simulink model "Vehicle"  (R2020a)
settings: Solver=VariableStepAuto  StartTime=0.0  StopTime=10.0  RelTol=1e-3
model workspace (MAT data in the model file):
  VEH.Mass = 330
  VEH.StaticNormalFrontLoad.FR = 74.25
  VEH.StaticNormalFrontLoad.FL = 74.25
  VEH.StaticNormalRearLoad.RR = 90.75
  VEH.StaticNormalRearLoad.RL = 90.75
  VEH.WheelBase = 1.575
  VEH.FrontAxlePositionfromCG = 0.847
  VEH.RearAxlePositionfromCG = 0.693
  VEH.HeightCG = 0.277
  VEH.FrontalArea = 1.435
  VEH.DragCoefficient = 0.33
  VEH.NumberOfWheelsPerAxle = 2
  VEH.Thread.FR = 1.705
  VEH.Thread.RR = 1.705
  VEH.PitchMomentInertia = 206
  VEH.RollMomentInertia = 206.613792
  VEH.YawMomentInertia = 206.613792
  VEH.SteeringRatio = 5.2
  VEH.TrackWidth = 1.2
  VEH.SprungMass = 290
  VEH.InitialLongPosition = 0
  VEH.InitialLatPosition = 0
  VEH.InitialVertPosition = 0
  VEH.InitialRollAngle = 0
  VEH.InitialPitchAngle = 0
  VEH.InitialYawAngle = 0
  VEH.InitialLongVel = 0
  VEH.InitialLatVel = 0
  VEH.InitialVertVel = 0
  VEH.InitialRollRate = 0
  VEH.InitialPitchRate = 0
  VEH.InitialYawRate = 0
  VEH.LongitudinalDragCoefficient = 1.06
  VEH.LongitudinalLCoefficient = -2.05
settings Model: Creator=Administrator  LastModifiedBy=Administrator

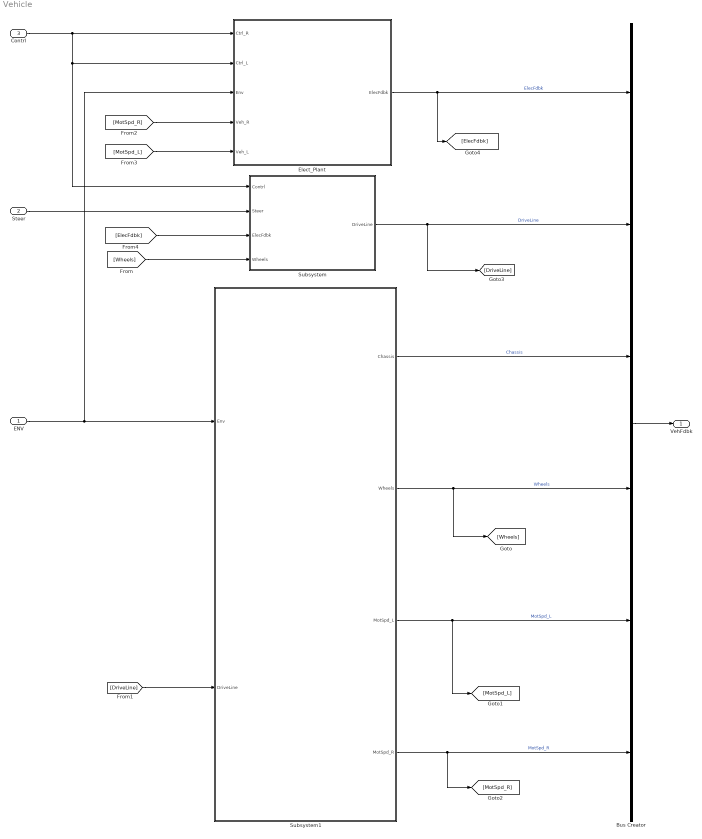
== system Vehicle ==
  ENV : Inport
  Steer : Inport  Port=2
  Contrl : Inport  Port=3
  Bus Creator : BusCreator  Inputs=6
  Elect_Plant : Subsystem
  Subsystem : Subsystem
  Subsystem1 : Subsystem
  VehFdbk : Outport  SignalName=VehFdbk
  wires:
  Elect_Plant/1(ElecFdbk) -> [ElecFdbk], Bus Creator/1  "ElecFdbk"
  Contrl/1 -> Elect_Plant/2(Ctrl_L), Subsystem/1(Contrl), Elect_Plant/1(Ctrl_R)
  Subsystem/1(DriveLine) -> [DriveLine], Bus Creator/2  "DriveLine"
  Subsystem1/1(Chassis) -> Bus Creator/3  "Chassis"
  Subsystem1/2(Wheels) -> [Wheels], Bus Creator/4  "Wheels"
  Subsystem1/3(MotSpd_L) -> [MotSpd_L], Bus Creator/5  "MotSpd_L"
  Subsystem1/4(MotSpd_R) -> [MotSpd_R], Bus Creator/6  "MotSpd_R"
  Bus Creator/1 -> VehFdbk/1
  [MotSpd_R] -> Elect_Plant/4(Veh_R)
  [MotSpd_L] -> Elect_Plant/5(Veh_L)
  Steer/1 -> Subsystem/2(Steer)
  [ElecFdbk] -> Subsystem/3(ElecFdbk)
  [Wheels] -> Subsystem/4(Wheels)
  ENV/1 -> Elect_Plant/3(Env), Subsystem1/1(Env)
  [DriveLine] -> Subsystem1/2(DriveLine)

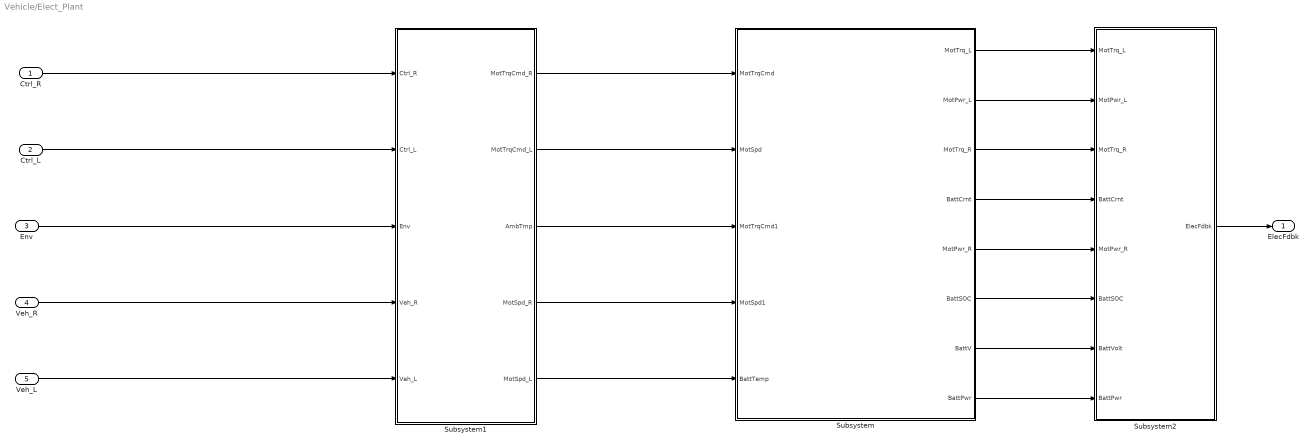
== system Vehicle/Elect_Plant ==
  Ctrl_R : Inport
  Ctrl_L : Inport  Port=2
  Env : Inport  Port=3
  Veh_R : Inport  Port=4
  Veh_L : Inport  Port=5
  Subsystem : Subsystem
  Subsystem1 : Subsystem
  Subsystem2 : Subsystem
  ElecFdbk : Outport
  wires:
  Subsystem1/4(MotSpd_R) -> Subsystem/4(MotSpd1)
  Subsystem1/1(MotTrqCmd_R) -> Subsystem/1(MotTrqCmd)
  Subsystem1/2(MotTrqCmd_L) -> Subsystem/2(MotSpd)
  Subsystem1/3(AmbTmp) -> Subsystem/3(MotTrqCmd1)
  Subsystem1/5(MotSpd_L) -> Subsystem/5(BattTemp)
  Veh_L/1 -> Subsystem1/5(Veh_L)
  Ctrl_R/1 -> Subsystem1/1(Ctrl_R)
  Ctrl_L/1 -> Subsystem1/2(Ctrl_L)
  Env/1 -> Subsystem1/3(Env)
  Veh_R/1 -> Subsystem1/4(Veh_R)
  Subsystem/1(MotTrq_L) -> Subsystem2/1(MotTrq_L)
  Subsystem/2(MotPwr_L) -> Subsystem2/2(MotPwr_L)
  Subsystem/3(MotTrq_R) -> Subsystem2/3(MotTrq_R)
  Subsystem/4(BattCrnt) -> Subsystem2/4(BattCrnt)
  Subsystem/5(MotPwr_R) -> Subsystem2/5(MotPwr_R)
  Subsystem/6(BattSOC) -> Subsystem2/6(BattSOC)
  Subsystem/7(BattV) -> Subsystem2/7(BattVolt)
  Subsystem/8(BattPwr) -> Subsystem2/8(BattPwr)
  Subsystem2/1(ElecFdbk) -> ElecFdbk/1

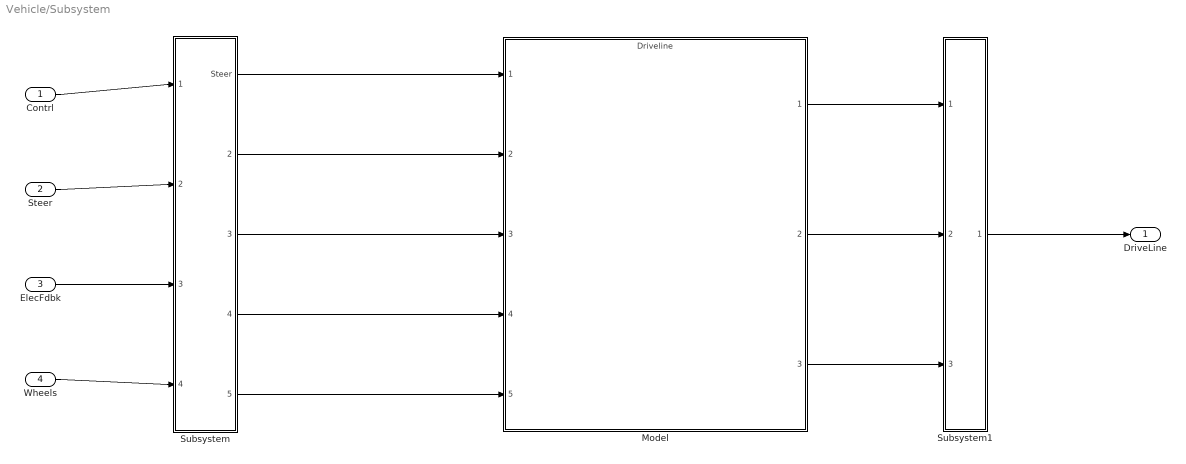
== system Vehicle/Subsystem ==
  Contrl : Inport
  Steer : Inport  Port=2
  ElecFdbk : Inport  Port=3
  Wheels : Inport  Port=4
  Model : ModelReference  ModelNameDialog=Driveline.slx  SimulationMode=Normal  ModelReferenceVersion=1.211
  Subsystem : Subsystem
  Subsystem1 : Subsystem
  DriveLine : Outport
  wires:
  Contrl/1 -> Subsystem/1(Contrl)
  Subsystem/1(Steer) -> Model/1
  Subsystem/2(MotTrq_L) -> Model/2
  Subsystem/3(MotTrq_R) -> Model/3
  Subsystem/4(PrsCmd) -> Model/4
  Subsystem/5(Omega) -> Model/5
  Steer/1 -> Subsystem/2(SteerCmd)
  Wheels/1 -> Subsystem/4(Wheels)
  ElecFdbk/1 -> Subsystem/3(ElecFdbk)
  Model/1 -> Subsystem1/1(WhlAng)
  Model/2 -> Subsystem1/2(AxlTrq)
  Model/3 -> Subsystem1/3(BrkPrs)
  Subsystem1/1(DriverLine) -> DriveLine/1

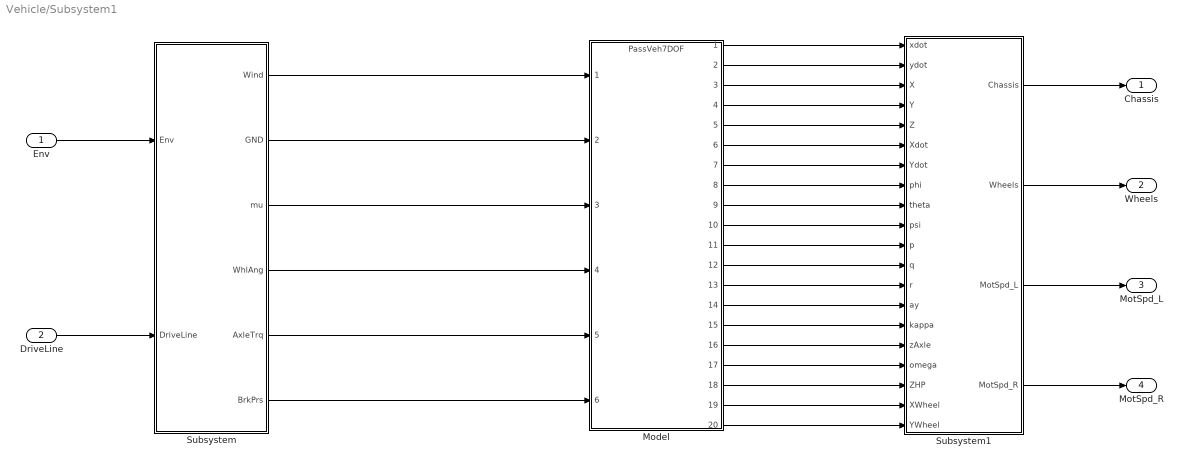
== system Vehicle/Subsystem1 ==
  Env : Inport
  DriveLine : Inport  Port=2
  Model : ModelReference  ModelNameDialog=PassVeh7DOF.slx  SimulationMode=Normal  ModelReferenceVersion=1.128
  Subsystem : Subsystem
  Subsystem1 : Subsystem
  Chassis : Outport
  Wheels : Outport  Port=2
  MotSpd_L : Outport  Port=3
  MotSpd_R : Outport  Port=4
  wires:
  Env/1 -> Subsystem/1(Env)
  Subsystem/1(Wind) -> Model/1
  Subsystem/2(GND) -> Model/2
  Subsystem/3(mu) -> Model/3
  Subsystem/4(WhlAng) -> Model/4
  Subsystem/5(AxleTrq) -> Model/5
  Subsystem/6(BrkPrs) -> Model/6
  DriveLine/1 -> Subsystem/2(DriveLine)
  Model/1 -> Subsystem1/1(xdot)
  Model/2 -> Subsystem1/2(ydot)
  Model/3 -> Subsystem1/3(X)
  Model/4 -> Subsystem1/4(Y)
  Model/5 -> Subsystem1/5(Z)
  Model/6 -> Subsystem1/6(Xdot)
  Model/7 -> Subsystem1/7(Ydot)
  Model/8 -> Subsystem1/8(phi)
  Model/9 -> Subsystem1/9(theta)
  Model/10 -> Subsystem1/10(psi)
  Model/11 -> Subsystem1/11(p)
  Model/12 -> Subsystem1/12(q)
  Model/13 -> Subsystem1/13(r)
  Model/14 -> Subsystem1/14(ay)
  Model/15 -> Subsystem1/15(kappa)
  Model/16 -> Subsystem1/16(zAxle)
  Model/17 -> Subsystem1/17(omega)
  Model/18 -> Subsystem1/18(ZHP)
  Model/19 -> Subsystem1/19(XWheel)
  Model/20 -> Subsystem1/20(YWheel)
  Subsystem1/1(Chassis) -> Chassis/1
  Subsystem1/2(Wheels) -> Wheels/1
  Subsystem1/3(MotSpd_L) -> MotSpd_L/1
  Subsystem1/4(MotSpd_R) -> MotSpd_R/1

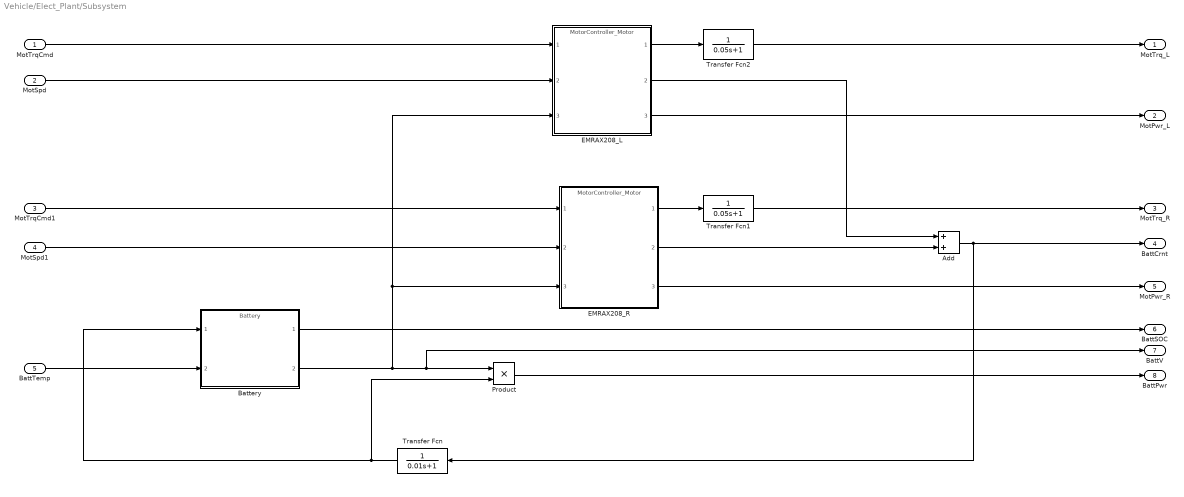
== system Vehicle/Elect_Plant/Subsystem ==
  MotTrqCmd : Inport
  MotSpd : Inport  Port=2
  MotTrqCmd1 : Inport  Port=3
  MotSpd1 : Inport  Port=4
  BattTemp : Inport  Port=5
  Add : Sum
  Battery : ModelReference  ModelNameDialog=Battery.slx  ModelReferenceVersion=1.1
  EMRAX208_L : ModelReference  ModelNameDialog=MotorController_Motor.slx  ModelReferenceVersion=1.1
  EMRAX208_R : ModelReference  ModelNameDialog=MotorController_Motor.slx  ModelReferenceVersion=1.1
  Product : Product
  Transfer Fcn : TransferFcn  Denominator=[0.01 1]
  Transfer Fcn1 : TransferFcn  Denominator=[0.05 1]
  Transfer Fcn2 : TransferFcn  Denominator=[0.05 1]
  MotTrq_L : Outport
  MotPwr_L : Outport  Port=2
  MotTrq_R : Outport  Port=3
  BattCrnt : Outport  Port=4
  MotPwr_R : Outport  Port=5
  BattSOC : Outport  Port=6
  BattV : Outport  Port=7
  BattPwr : Outport  Port=8
  wires:
  Transfer Fcn/1 -> Product/2, Battery/1
  MotTrqCmd/1 -> EMRAX208_L/1
  EMRAX208_R/2 -> Add/2
  EMRAX208_R/3 -> MotPwr_R/1
  Add/1 -> BattCrnt/1, Transfer Fcn/1
  Battery/1 -> BattSOC/1
  EMRAX208_L/1 -> Transfer Fcn2/1
  Transfer Fcn2/1 -> MotTrq_L/1
  EMRAX208_L/2 -> Add/1
  MotSpd1/1 -> EMRAX208_R/2
  Battery/2 -> EMRAX208_R/3, EMRAX208_L/3, BattV/1, Product/1
  EMRAX208_R/1 -> Transfer Fcn1/1
  EMRAX208_L/3 -> MotPwr_L/1
  Transfer Fcn1/1 -> MotTrq_R/1
  MotSpd/1 -> EMRAX208_L/2
  BattTemp/1 -> Battery/2
  MotTrqCmd1/1 -> EMRAX208_R/1
  Product/1 -> BattPwr/1

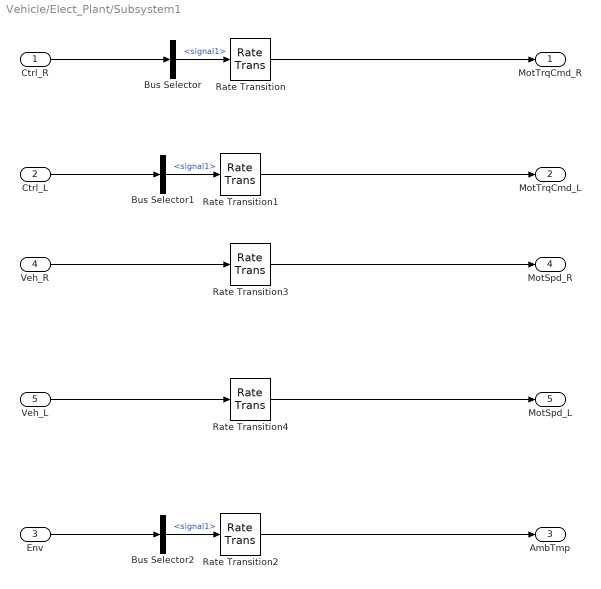
== system Vehicle/Elect_Plant/Subsystem1 ==
  Ctrl_R : Inport
  Ctrl_L : Inport  Port=2
  Env : Inport  Port=3
  Veh_R : Inport  Port=4
  Veh_L : Inport  Port=5
  Bus Selector : BusSelector  OutputSignals=signal1
  Bus Selector1 : BusSelector  OutputSignals=signal1
  Bus Selector2 : BusSelector  OutputSignals=signal1
  Rate Transition : RateTransition  Deterministic=off
  Rate Transition{1..4} (4 alike) : RateTransition
  MotTrqCmd_R : Outport
  MotTrqCmd_L : Outport  Port=2
  AmbTmp : Outport  Port=3
  MotSpd_R : Outport  Port=4
  MotSpd_L : Outport  Port=5
  wires:
  Bus Selector/1 -> Rate Transition/1  "<signal1>"
  Rate Transition/1 -> MotTrqCmd_R/1
  Ctrl_R/1 -> Bus Selector/1
  Ctrl_L/1 -> Bus Selector1/1
  Rate Transition1/1 -> MotTrqCmd_L/1
  Bus Selector1/1 -> Rate Transition1/1  "<signal1>"
  Bus Selector2/1 -> Rate Transition2/1  "<signal1>"
  Rate Transition2/1 -> AmbTmp/1
  Env/1 -> Bus Selector2/1
  Veh_L/1 -> Rate Transition4/1
  Veh_R/1 -> Rate Transition3/1
  Rate Transition4/1 -> MotSpd_L/1
  Rate Transition3/1 -> MotSpd_R/1

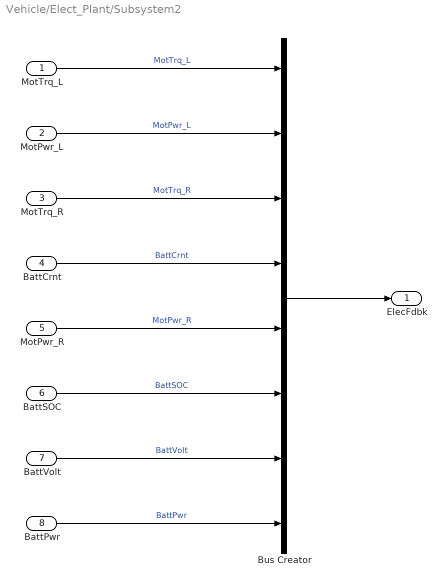
== system Vehicle/Elect_Plant/Subsystem2 ==
  MotTrq_L : Inport
  MotPwr_L : Inport  Port=2
  MotTrq_R : Inport  Port=3
  BattCrnt : Inport  Port=4
  MotPwr_R : Inport  Port=5
  BattSOC : Inport  Port=6
  BattVolt : Inport  Port=7
  BattPwr : Inport  Port=8
  Bus Creator : BusCreator  Inputs=8
  ElecFdbk : Outport
  wires:
  MotPwr_R/1 -> Bus Creator/5  "MotPwr_R"
  BattCrnt/1 -> Bus Creator/4  "BattCrnt"
  Bus Creator/1 -> ElecFdbk/1
  MotTrq_R/1 -> Bus Creator/3  "MotTrq_R"
  MotPwr_L/1 -> Bus Creator/2  "MotPwr_L"
  BattVolt/1 -> Bus Creator/7  "BattVolt"
  MotTrq_L/1 -> Bus Creator/1  "MotTrq_L"
  BattPwr/1 -> Bus Creator/8  "BattPwr"
  BattSOC/1 -> Bus Creator/6  "BattSOC"

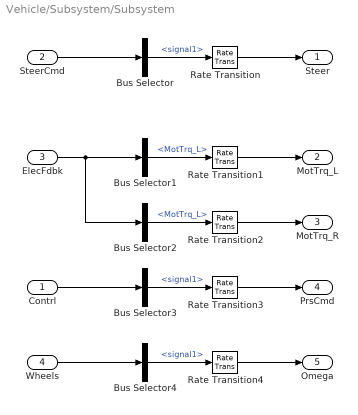
== system Vehicle/Subsystem/Subsystem ==
  Contrl : Inport
  SteerCmd : Inport  Port=2
  ElecFdbk : Inport  Port=3
  Wheels : Inport  Port=4
  Bus Selector : BusSelector  OutputSignals=signal1
  Bus Selector1 : BusSelector  OutputSignals=MotTrq_L
  Bus Selector2 : BusSelector  OutputSignals=MotTrq_L
  Bus Selector3 : BusSelector  OutputSignals=signal1
  Bus Selector4 : BusSelector  OutputSignals=signal1
  Rate Transition{,1..4} (5 alike) : RateTransition
  Steer : Outport
  MotTrq_L : Outport  Port=2
  MotTrq_R : Outport  Port=3
  PrsCmd : Outport  Port=4
  Omega : Outport  Port=5
  wires:
  Bus Selector/1 -> Rate Transition/1  "<signal1>"
  SteerCmd/1 -> Bus Selector/1
  ElecFdbk/1 -> Bus Selector2/1, Bus Selector1/1
  Wheels/1 -> Bus Selector4/1
  Bus Selector4/1 -> Rate Transition4/1  "<signal1>"
  Bus Selector3/1 -> Rate Transition3/1  "<signal1>"
  Contrl/1 -> Bus Selector3/1
  Bus Selector1/1 -> Rate Transition1/1  "<MotTrq_L>"
  Bus Selector2/1 -> Rate Transition2/1  "<MotTrq_L>"
  Rate Transition/1 -> Steer/1
  Rate Transition1/1 -> MotTrq_L/1
  Rate Transition2/1 -> MotTrq_R/1
  Rate Transition3/1 -> PrsCmd/1
  Rate Transition4/1 -> Omega/1

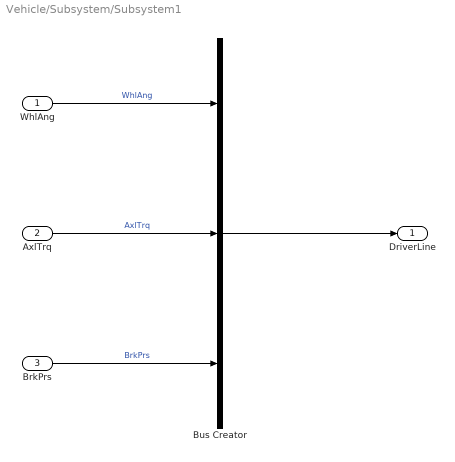
== system Vehicle/Subsystem/Subsystem1 ==
  WhlAng : Inport
  AxlTrq : Inport  Port=2
  BrkPrs : Inport  Port=3
  Bus Creator : BusCreator  Inputs=3
  DriverLine : Outport
  wires:
  AxlTrq/1 -> Bus Creator/2  "AxlTrq"
  WhlAng/1 -> Bus Creator/1  "WhlAng"
  BrkPrs/1 -> Bus Creator/3  "BrkPrs"
  Bus Creator/1 -> DriverLine/1

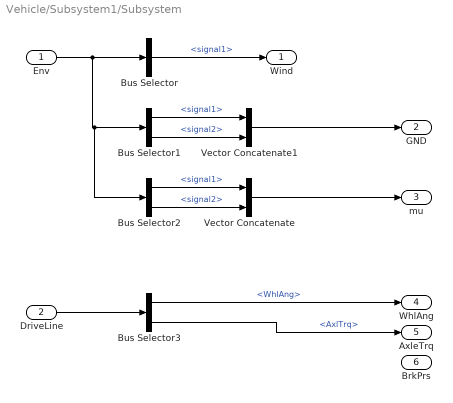
== system Vehicle/Subsystem1/Subsystem ==
  Env : Inport
  DriveLine : Inport  Port=2
  Bus Selector : BusSelector  OutputSignals=signal1
  Bus Selector1 : BusSelector  OutputSignals=signal1,signal2
  Bus Selector2 : BusSelector  OutputSignals=signal1,signal2
  Bus Selector3 : BusSelector  OutputSignals=WhlAng,AxlTrq
  Vector Concatenate : Concatenate
  Vector Concatenate1 : Concatenate
  Wind : Outport
  GND : Outport  Port=2
  mu : Outport  Port=3
  WhlAng : Outport  Port=4
  AxleTrq : Outport  Port=5
  BrkPrs : Outport  Port=6
  wires:
  Bus Selector/1 -> Wind/1  "<signal1>"
  Env/1 -> Bus Selector2/1, Bus Selector1/1, Bus Selector/1
  Bus Selector2/2 -> Vector Concatenate/2  "<signal2>"
  Vector Concatenate/1 -> mu/1
  Bus Selector2/1 -> Vector Concatenate/1  "<signal1>"
  Bus Selector1/1 -> Vector Concatenate1/1  "<signal1>"
  Bus Selector1/2 -> Vector Concatenate1/2  "<signal2>"
  Vector Concatenate1/1 -> GND/1
  DriveLine/1 -> Bus Selector3/1
  Bus Selector3/1 -> WhlAng/1  "<WhlAng>"
  Bus Selector3/2 -> AxleTrq/1  "<AxlTrq>"

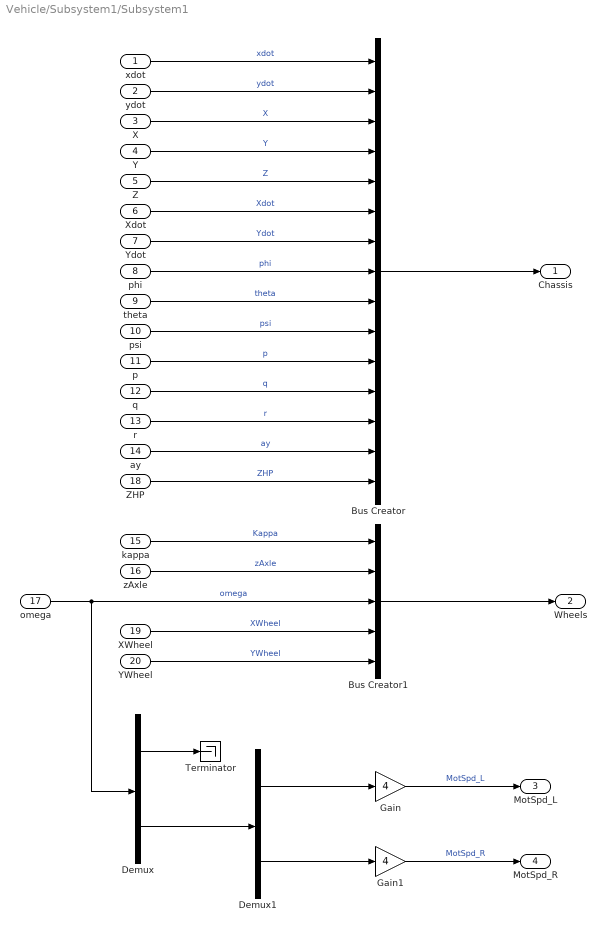
== system Vehicle/Subsystem1/Subsystem1 ==
  xdot : Inport
  ydot : Inport  Port=2
  X : Inport  Port=3
  Y : Inport  Port=4
  Z : Inport  Port=5
  Xdot : Inport  Port=6
  Ydot : Inport  Port=7
  phi : Inport  Port=8
  theta : Inport  Port=9
  psi : Inport  Port=10
  p : Inport  Port=11
  q : Inport  Port=12
  r : Inport  Port=13
  ay : Inport  Port=14
  kappa : Inport  Port=15
  zAxle : Inport  Port=16
  omega : Inport  Port=17
  ZHP : Inport  Port=18
  XWheel : Inport  Port=19
  YWheel : Inport  Port=20
  Bus Creator : BusCreator  Inputs=15
  Bus Creator1 : BusCreator  Inputs=5
  Demux : Demux  Outputs=2
  Demux1 : Demux  Outputs=2
  Gain : Gain  Gain=4
  Gain1 : Gain  Gain=4
  Terminator : Terminator
  Chassis : Outport
  Wheels : Outport  Port=2
  MotSpd_L : Outport  Port=3
  MotSpd_R : Outport  Port=4
  wires:
  Y/1 -> Bus Creator/4  "Y"
  Bus Creator/1 -> Chassis/1
  xdot/1 -> Bus Creator/1  "xdot"
  phi/1 -> Bus Creator/8  "phi"
  ydot/1 -> Bus Creator/2  "ydot"
  theta/1 -> Bus Creator/9  "theta"
  Xdot/1 -> Bus Creator/6  "Xdot"
  Z/1 -> Bus Creator/5  "Z"
  X/1 -> Bus Creator/3  "X"
  Ydot/1 -> Bus Creator/7  "Ydot"
  psi/1 -> Bus Creator/10  "psi"
  ay/1 -> Bus Creator/14  "ay"
  p/1 -> Bus Creator/11  "p"
  r/1 -> Bus Creator/13  "r"
  q/1 -> Bus Creator/12  "q"
  ZHP/1 -> Bus Creator/15  "ZHP"
  kappa/1 -> Bus Creator1/1  "Kappa"
  zAxle/1 -> Bus Creator1/2  "zAxle"
  omega/1 -> Demux/1, Bus Creator1/3  "omega"
  XWheel/1 -> Bus Creator1/4  "XWheel"
  YWheel/1 -> Bus Creator1/5  "YWheel"
  Demux/1 -> Terminator/1
  Demux/2 -> Demux1/1
  Demux1/1 -> Gain/1
  Demux1/2 -> Gain1/1
  Bus Creator1/1 -> Wheels/1
  Gain1/1 -> MotSpd_R/1  "MotSpd_R"
  Gain/1 -> MotSpd_L/1  "MotSpd_L"
